simulink model "hitsi3_injector_circuits (1)"  (R2019a)
settings: Solver=VariableStepAuto  StartTime=0.0  StopTime=5e-3  RelTol=1e-3
undefined symbols (not defined in the file or in its folder): K, sysC, sysKf, Vspa
settings Model: Creator=akaptano  LastModifiedBy=akaptano

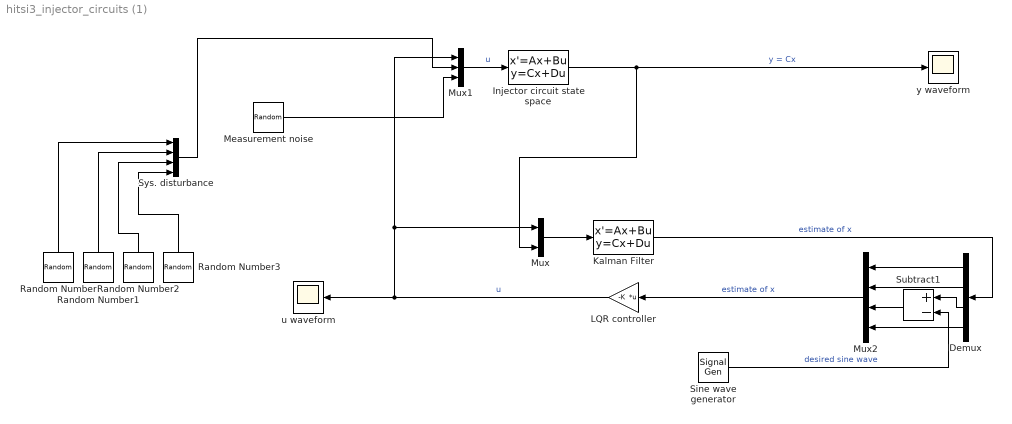
== system hitsi3_injector_circuits (1) ==
  Demux : Demux
  Injector circuit state space : StateSpace  A=sysC.a  B=sysC.b  C=sysC.c  D=sysC.d  InitialCondition=[0 0 0 0]
  Kalman Filter : StateSpace  A=sysKf.a  B=sysKf.b  C=sysKf.c  D=sysKf.d  InitialCondition=[0 0 0 0]
  LQR controller : Gain  Gain=-K  Multiplication=Matrix(K*u) (u vector)
  Measurement noise : RandomNumber  SampleTime=0.1
  Mux : Mux  Inputs=2
  Mux1 : Mux  Inputs=3
  Mux2 : Mux
  Random Number{,1..3} (4 alike) : RandomNumber  SampleTime=0.1
  Sine wave generator : SignalGenerator  Amplitude=Vspa  Frequency=14500
  Subtract1 : Sum  Inputs=+-
  Sys. disturbance : Mux
  u waveform : Scope
  y waveform : Scope
  wires:
  Mux/1 -> Kalman Filter/1
  Mux1/1 -> Injector circuit state space/1  "u"
  Measurement noise/1 -> Mux1/3
  Random Number3/1 -> Sys. disturbance/4
  Random Number2/1 -> Sys. disturbance/3
  Random Number1/1 -> Sys. disturbance/2
  Random Number/1 -> Sys. disturbance/1
  Sys. disturbance/1 -> Mux1/2
  Mux2/1 -> LQR controller/1  "estimate of x"
  Demux/4 -> Mux2/4
  Demux/2 -> Mux2/2
  Demux/1 -> Mux2/1
  Kalman Filter/1 -> Demux/1  "estimate of x"
  Demux/3 -> Subtract1/1
  Subtract1/1 -> Mux2/3
  Sine wave generator/1 -> Subtract1/2  "desired sine wave"
  Injector circuit state space/1 -> y waveform/1, Mux/2  "y = Cx"
  LQR controller/1 -> u waveform/1, Mux1/1, Mux/1  "u"
